simulink model "trial1"  (R2022a)
settings: Solver=VariableStepAuto  StartTime=0.0  StopTime=10.0  RelTol=1e-3
libraries: spsSeriesRLCBranchLib x6, spsVoltageMeasurementLib x6, spsDiodeLib x2, spsGroundLib x2, spsMosfetLib x2, spsDCVoltageSourceLib x1, spsPVArrayLib x1, eePwmGenerator x1, spsSeriesRLCLoadLib x1, spspowerguiLib x1
settings Model: Creator=baikhyeongmeon  LastModifiedBy=baikhyeongmeon

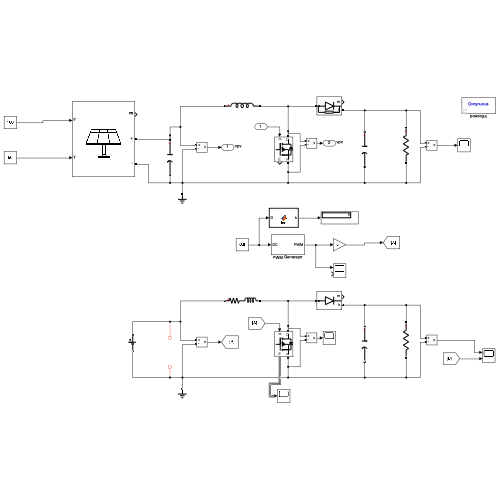
[thumbnail: Simulink's stored preview of the top-level diagram]
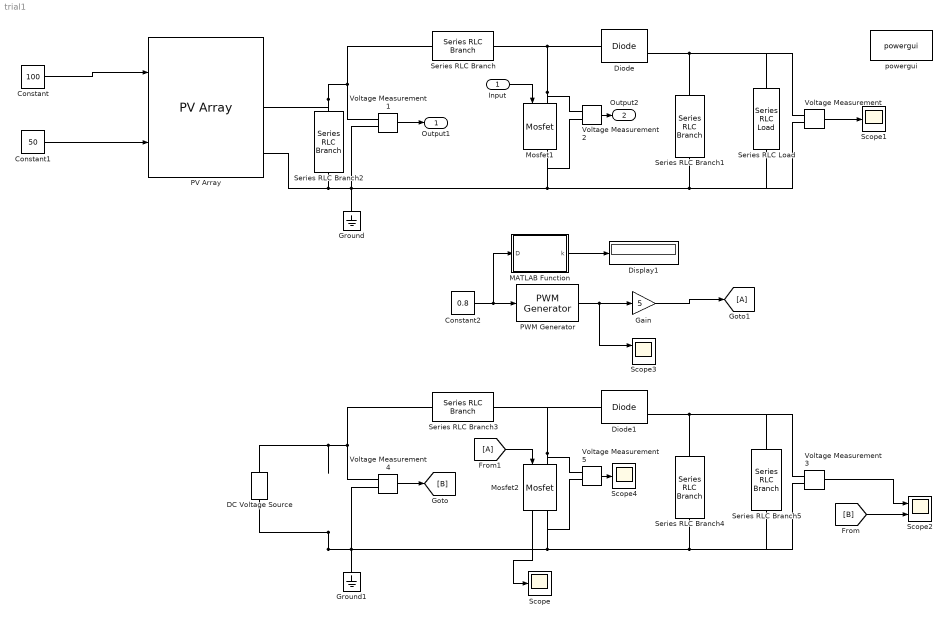
== system trial1 ==
  Input : Inport
  Constant : Constant  Value=100
  Constant1 : Constant  Value=50
  Constant2 : Constant  Value=0.8
  DC Voltage Source : spsDCVoltageSourceLib/DC Voltage Source  Amplitude=50  Measurements=None
  Diode : spsDiodeLib/Diode  Ron=0.001  Lon=0  Vf=0.8  IC=0  UseSnubber=0  Rs=500  Cs=250e-9  Measurements=on
  Diode1 : spsDiodeLib/Diode  Ron=0  Lon=0  Vf=0.8  IC=0  UseSnubber=0  Rs=0  Cs=0  Measurements=on
  Display1 : Display
  From1 : From
  Gain : Gain  Gain=5
  Goto1 : Goto
  Ground : spsGroundLib/Ground  LConnTagsString=a
  Ground1 : spsGroundLib/Ground  LConnTagsString=a
  MATLAB Function : MATLAB Function  TreatAsAtomicUnit=on
  Mosfet1 : spsMosfetLib/Mosfet  Ron=0.1  Lon=0  Rd=0.01  Vfd=0  IC=0  Rs=1e5  Cs=inf  Measurements=on
  Mosfet2 : spsMosfetLib/Mosfet  Ron=0.1  Lon=0  Rd=0.01  Vfd=0  IC=0  Rs=0  Cs=0  Measurements=on
  PV Array : spsPVArrayLib/PV Array  Npar=40  Nser=10  PlotType=array @ 1000 W/m2 & specified temperatures  S_vec="[ 1000  500  100 ]"  Temp_C_vec="[ 45 25  ]"  ModuleName=User-defined  PlotWhenSelected=off  Pm=213.15  Ncell=60  Voc=36.3  Isc=7.84  Vm=29  Im=7.35  beta_Voc_pc=-0.36099  alpha_Isc_pc=0.102  beta_Voc=-0.13104  alpha_Isc=0.0079968  IL=7.8654  I0=2.9273e-10  nI=0.98119  Rsh=313.0553  Rs=0.39381  RobustModel=off  RobustCellTemperature=313.3991  BAL=on  Tc=1e-6  Tfilter=5e-5
  PWM Generator : eePwmGenerator/PWM Generator  CarrCount=Up  Tper=0.01  Tdelay=0  Ts=5e-5
  Scope : Scope
  Scope1 : Scope
  Scope2 : Scope  NumInputPorts=2
  Scope3 : Scope  NumInputPorts=2
  Scope4 : Scope
  Series RLC Branch : spsSeriesRLCBranchLib/Series RLC Branch  LConnTagsString=__new0  RConnTagsString=__new0  BranchType=L  Resistance=1  Inductance=1e-3  SetiL0=off  InitialCurrent=0  Capacitance=1e-6  Setx0=off  InitialVoltage=0  Measurements=None
  Series RLC Branch1 : spsSeriesRLCBranchLib/Series RLC Branch  LConnTagsString=__new0  RConnTagsString=__new0  BranchType=C  Resistance=1  Inductance=1e-3  SetiL0=off  InitialCurrent=0  Capacitance=1e-6  Setx0=off  InitialVoltage=0  Measurements=None
  Series RLC Branch2 : spsSeriesRLCBranchLib/Series RLC Branch  LConnTagsString=__new0  RConnTagsString=__new0  BranchType=C  Resistance=1  Inductance=1e-3  SetiL0=off  InitialCurrent=0  Capacitance=1e-6  Setx0=off  InitialVoltage=0  Measurements=None
  Series RLC Branch3 : spsSeriesRLCBranchLib/Series RLC Branch  LConnTagsString=__new0  RConnTagsString=__new0  BranchType=RL  Resistance=10e-3  Inductance=1e-4  SetiL0=off  InitialCurrent=0  Capacitance=1e-6  Setx0=off  InitialVoltage=0  Measurements=None
  Series RLC Branch4 : spsSeriesRLCBranchLib/Series RLC Branch  LConnTagsString=__new0  RConnTagsString=__new0  BranchType=C  Resistance=1  Inductance=1e-3  SetiL0=off  InitialCurrent=0  Capacitance=10e-3  Setx0=off  InitialVoltage=0  Measurements=None
  Series RLC Branch5 : spsSeriesRLCBranchLib/Series RLC Branch  LConnTagsString=__new0  RConnTagsString=__new0  BranchType=R  Resistance=10  Inductance=1e-3  SetiL0=off  InitialCurrent=0  Capacitance=1e-6  Setx0=off  InitialVoltage=0  Measurements=None
  Series RLC Load : spsSeriesRLCLoadLib/Series RLC Load  LConnTagsString=a  RConnTagsString=__new0  NominalVoltage=1000  NominalFrequency=60  ActivePower=10e3  InductivePower=0  CapacitivePower=0  Setx0=off  InitialVoltage=0  SetiL0=off  InitialCurrent=0  Measurements=None  LoadType=constant Z
  Voltage Measurement{,1..5} (6 alike) : spsVoltageMeasurementLib/Voltage Measurement  PhasorSimulation=off  OutputType=Complex  PSBequivalent=0
  powergui : spspowerguiLib/powergui  Priority=1  SimulationMode=Continuous  SampleTime=50e-6  frequency=60  Iterations=50  frequencyindice=0  Pbase=100e6  ErrMax=1e-4  UnitsV=kV  UnitsW=MW  buscounter=0  FunctionMessages=off  echomessages=off  EnableUseOfTLC=off  CurrentSourceSwitches=off  DisableSnubberDevices=off  DisableRonSwitches=off  DisableVfSwitches=off  DisplayEquations=off  AutomaticDiscreteSolvers=off  SolverType=Tustin/Backward Euler (TBE)  Interpol=off  ExternalGateDelay=off  methode=off  Ts=100  x0status=blocks  SPID=on  SwTol=0  HookPort=off  NonlinearTolerance=1e-4  nMaxIteration=100  ContinueOnMaxIteration=off  RestoreLinks=warning  ResistiveCurrentMeasurement=off  Frange=[0:2:500]  Ylog=off  Xlog=on  ShowGrid=off  save=off  variable=ZData  structure=0  ZoomFFT=off  StartTime=0.0  cycles=1  DisplayStyle=1  fundamental=60  FreqAxis=off  MaxFrequency=1000  frequencyindicesteady=1  RmsSteady=1  display=off
  Output1 : Outport  SignalName=vpv
  Output2 : Outport  Port=2  SignalName=vpv
  wires:
  Input/1 -> Mosfet1/1
  Constant/1 -> PV Array/1
  Constant1/1 -> PV Array/2
  Constant2/1 -> MATLAB Function/1(D), PWM Generator/1
  PWM Generator/1 -> Gain/1, Scope3/1
  Voltage Measurement/1 -> Scope1/1
  Voltage Measurement1/1 -> Output1/1
  Voltage Measurement2/1 -> Output2/1
  Voltage Measurement4/1 -> [B]
  Voltage Measurement3/1 -> Scope2/1
  Voltage Measurement5/1 -> Scope4/1
  From1/1 -> Mosfet2/1
  [B] -> Scope2/2
  Gain/1 -> Goto1/1
  Mosfet2/1 -> Scope/1
  MATLAB Function/1(k) -> Display1/1
  connections:
  PV Array/RConn1 -- Series RLC Branch2/LConn1 -- Series RLC Branch/LConn1 -- Voltage Measurement1/LConn1
  PV Array/RConn2 -- Voltage Measurement1/LConn2 -- Voltage Measurement2/LConn2 -- Mosfet1/RConn1 -- Series RLC Load/RConn1 -- Voltage Measurement/LConn2 -- Series RLC Branch1/RConn1 -- Ground/LConn1 -- Series RLC Branch2/RConn1
  Series RLC Branch/RConn1 -- Voltage Measurement2/LConn1 -- Mosfet1/LConn1 -- Diode/LConn1
  Diode/RConn1 -- Series RLC Load/LConn1 -- Voltage Measurement/LConn1 -- Series RLC Branch1/LConn1
  DC Voltage Source/LConn1 -- Voltage Measurement4/LConn2 -- Voltage Measurement5/LConn2 -- Mosfet2/RConn1 -- Series RLC Branch5/RConn1 -- Voltage Measurement3/LConn2 -- Series RLC Branch4/RConn1 -- Ground1/LConn1
  Mosfet2/LConn1 -- Series RLC Branch3/RConn1 -- Diode1/LConn1 -- Voltage Measurement5/LConn1
  Diode1/RConn1 -- Series RLC Branch4/LConn1 -- Series RLC Branch5/LConn1 -- Voltage Measurement3/LConn1
  DC Voltage Source/RConn1 -- Series RLC Branch3/LConn1 -- Voltage Measurement4/LConn1

== matlab function trial1/MATLAB Function ==
  data: D input; k output
function k = fcn(D)

k = 1/(1-D);
